simulink model "SF049A_LoaMgr"  (R2013b)
settings: Solver=FixedStepDiscrete  SolverMode=SingleTasking  StartTime=0.0  StopTime=1  FixedStep=0.002  RelTol=1e-3
undefined symbols (not defined in the file): CURRMEASLOAMTGTNMASK_CNT_U08, IVTRLOAMTGTNMASK_CNT_U08, LoaCtrldShtdwn, LoaCurrMeasIdptSigNrFlt, LoaHwTqIdptSigNrFlt, LoaImdtShtdwn, LoaIvtrIdptSigNrFlt, LOAMAXSLEW_ULSPERSEC_F32, LoaMgrCurrIvtrMtgtnRate, LoaMgrCurrIvtrMtgtnSca, LoaMgrCurrIvtrMtgtnScaZeroEna, LoaMgrCurrMeasIdptSig0Resp, LoaMgrCurrMeasIdptSig1Resp, LoaMgrCurrMeasIdptSig2Resp, LoaMgrCurrMeasIdptSigFltThd, LoaMgrCurrMeasMtgtnRate, LoaMgrCurrMeasMtgtnSca, LoaMgrCurrMeasMtgtnScaZeroEna, LoaMgrFadeOutStRate, LoaMgrHwTqIdptSig0NoTqLoaResp, LoaMgrHwTqIdptSig1NoTqLoaResp, LoaMgrHwTqIdptSig2Resp, LoaMgrHwTqIdptSig4Resp, LoaMgrHwTqIdptSigFltThd, LoaMgrHwTqLoaAvlResp, LoaMgrIvtrIdptSig0Resp, LoaMgrIvtrIdptSig1Resp, LoaMgrIvtrIdptSig2Resp, LoaMgrIvtrIdptSigFltThd, LoaMgrIvtrMtgtnRate, LoaMgrIvtrMtgtnSca, LoaMgrIvtrMtgtnScaZeroEna, LoaMgrLimdStRate, LoaMgrLimdStSca, LoaMgrMotAgAvlSnsrlsResp, LoaMgrMotAgIdptSig0NoSnsrlsResp, LoaMgrMotAgIdptSig1NoSnsrlsResp, LoaMgrMotAgIdptSig2Resp, LoaMgrMotAgIdptSig3Resp, LoaMgrMotAgIdptSigFltThd, LoaMgrMotAgMtgtnRate, LoaMgrMotAgMtgtnSca, LoaMgrMotAgMtgtnScaZeroEna, LoaMotAgIdptSigNrFlt, LOASCAONE_ULS_F32, LOASCAZERO_ULS_F32, LoaSt1, LOASTIMDTSHTDWN_CNT_U08, LOASTNORM_CNT_U08, LOASTSWMTGTN_CNT_U08, MAXCURRMEASIDPTSIGALLWD_CNT_U08, MAXHWTQIDPTSIGALLWD_CNT_U08, MAXIVTRIDPTSIGALLWD_CNT_U08, MAXMOTAGMECLIDPTSIGALLWD_CNT_U08, NODEBSTEP_CNT_U16, NtcSts1, SigQlfr1
libraries: simulink x30, NxtrMin x4, NxtrMax x4, NxtrLim x2
(part 7 of 7)

== system SF049A_LoaMgr/LoaMgr/LoaMgrPer1/Request_Responses/HwTqResp/Zero_or_Invalid/cal1 ==
  In1 : Inport
  Action Port : ActionPort  ActionType=then
  CopyRight2 : Subsystem  Description=|  mask(Copyright Information){none=on}
      | Copyright info block.                                               
      |                                                                     
      | Place copyright information at the top of every subsystem in design.
      mask prompts: none "No parameters"
      mask help: Place copyright information at the top of every subsystem in design.
      mask Display:
      | NxtrConf = 'Nexteer Confidential';
      | 
      | sys = bdroot; %handle for the current model ("system")
      | first = get_param(sys,'Created');
      | first = first(end-3:end);  %year is last four digits
      | 
      | last = get_param(sys,'LastModifiedDate');
      | if isempty(last)
      |     last = datestr(now,'yyyy');
      | else
      |     last = last(end-3:end);
      | end
      | 
      | if strcmp(first,last)
      |     fprintf('%s -- Copyright %s Nexteer',NxtrConf,first)
      | else
      |     fprintf('%s -- %s%s- %s Nexteer',NxtrConf,char(169),first,last)
      | end
  Out2 : Outport
  wires:
  In1/1 -> Out2/1

== system SF049A_LoaMgr/LoaMgr/LoaMgrPer1/Request_Responses/HwTqResp/Zero_or_Invalid/cal2 ==
  In1 : Inport
  Action Port : ActionPort  ActionType=else
  CopyRight2 : Subsystem  Description=|  mask(Copyright Information){none=on}
      | Copyright info block.                                               
      |                                                                     
      | Place copyright information at the top of every subsystem in design.
      mask prompts: none "No parameters"
      mask help: Place copyright information at the top of every subsystem in design.
      mask Display:
      | NxtrConf = 'Nexteer Confidential';
      | 
      | sys = bdroot; %handle for the current model ("system")
      | first = get_param(sys,'Created');
      | first = first(end-3:end);  %year is last four digits
      | 
      | last = get_param(sys,'LastModifiedDate');
      | if isempty(last)
      |     last = datestr(now,'yyyy');
      | else
      |     last = last(end-3:end);
      | end
      | 
      | if strcmp(first,last)
      |     fprintf('%s -- Copyright %s Nexteer',NxtrConf,first)
      | else
      |     fprintf('%s -- %s%s- %s Nexteer',NxtrConf,char(169),first,last)
      | end
  Out1 : Outport
  wires:
  In1/1 -> Out1/1

== system SF049A_LoaMgr/LoaMgr/LoaMgrPer1/Request_Responses/HwTqResp/one/CopyRight2 ==

== system SF049A_LoaMgr/LoaMgr/LoaMgrPer1/Request_Responses/HwTqResp/one/cal1 ==
  In1 : Inport
  Action Port : ActionPort  ActionType=then
  CopyRight2 : Subsystem  Description=|  mask(Copyright Information){none=on}
      | Copyright info block.                                               
      |                                                                     
      | Place copyright information at the top of every subsystem in design.
      mask prompts: none "No parameters"
      mask help: Place copyright information at the top of every subsystem in design.
      mask Display:
      | NxtrConf = 'Nexteer Confidential';
      | 
      | sys = bdroot; %handle for the current model ("system")
      | first = get_param(sys,'Created');
      | first = first(end-3:end);  %year is last four digits
      | 
      | last = get_param(sys,'LastModifiedDate');
      | if isempty(last)
      |     last = datestr(now,'yyyy');
      | else
      |     last = last(end-3:end);
      | end
      | 
      | if strcmp(first,last)
      |     fprintf('%s -- Copyright %s Nexteer',NxtrConf,first)
      | else
      |     fprintf('%s -- %s%s- %s Nexteer',NxtrConf,char(169),first,last)
      | end
  Out2 : Outport
  wires:
  In1/1 -> Out2/1

== system SF049A_LoaMgr/LoaMgr/LoaMgrPer1/Request_Responses/HwTqResp/one/cal2 ==
  In1 : Inport
  Action Port : ActionPort  ActionType=else
  CopyRight2 : Subsystem  Description=|  mask(Copyright Information){none=on}
      | Copyright info block.                                               
      |                                                                     
      | Place copyright information at the top of every subsystem in design.
      mask prompts: none "No parameters"
      mask help: Place copyright information at the top of every subsystem in design.
      mask Display:
      | NxtrConf = 'Nexteer Confidential';
      | 
      | sys = bdroot; %handle for the current model ("system")
      | first = get_param(sys,'Created');
      | first = first(end-3:end);  %year is last four digits
      | 
      | last = get_param(sys,'LastModifiedDate');
      | if isempty(last)
      |     last = datestr(now,'yyyy');
      | else
      |     last = last(end-3:end);
      | end
      | 
      | if strcmp(first,last)
      |     fprintf('%s -- Copyright %s Nexteer',NxtrConf,first)
      | else
      |     fprintf('%s -- %s%s- %s Nexteer',NxtrConf,char(169),first,last)
      | end
  Out1 : Outport
  wires:
  In1/1 -> Out1/1

== system SF049A_LoaMgr/LoaMgr/LoaMgrPer1/Request_Responses/InvtrResp/Two/CopyRight2 ==

== system SF049A_LoaMgr/LoaMgr/LoaMgrPer1/Request_Responses/InvtrResp/Zero_or_Invalid/CopyRight2 ==

== system SF049A_LoaMgr/LoaMgr/LoaMgrPer1/Request_Responses/InvtrResp/one/CopyRight2 ==

== system SF049A_LoaMgr/LoaMgr/LoaMgrPer1/Request_Responses/MotAgResp/Three/CopyRight2 ==

== system SF049A_LoaMgr/LoaMgr/LoaMgrPer1/Request_Responses/MotAgResp/Two/CopyRight2 ==

== system SF049A_LoaMgr/LoaMgr/LoaMgrPer1/Request_Responses/MotAgResp/Zero_or_Invalid/CopyRight2 ==

== system SF049A_LoaMgr/LoaMgr/LoaMgrPer1/Request_Responses/MotAgResp/Zero_or_Invalid/cal1 ==
  In1 : Inport
  Action Port : ActionPort  ActionType=then
  CopyRight2 : Subsystem  Description=|  mask(Copyright Information){none=on}
      | Copyright info block.                                               
      |                                                                     
      | Place copyright information at the top of every subsystem in design.
      mask prompts: none "No parameters"
      mask help: Place copyright information at the top of every subsystem in design.
      mask Display:
      | NxtrConf = 'Nexteer Confidential';
      | 
      | sys = bdroot; %handle for the current model ("system")
      | first = get_param(sys,'Created');
      | first = first(end-3:end);  %year is last four digits
      | 
      | last = get_param(sys,'LastModifiedDate');
      | if isempty(last)
      |     last = datestr(now,'yyyy');
      | else
      |     last = last(end-3:end);
      | end
      | 
      | if strcmp(first,last)
      |     fprintf('%s -- Copyright %s Nexteer',NxtrConf,first)
      | else
      |     fprintf('%s -- %s%s- %s Nexteer',NxtrConf,char(169),first,last)
      | end
  Out2 : Outport
  wires:
  In1/1 -> Out2/1

== system SF049A_LoaMgr/LoaMgr/LoaMgrPer1/Request_Responses/MotAgResp/Zero_or_Invalid/cal2 ==
  In1 : Inport
  Action Port : ActionPort  ActionType=else
  CopyRight2 : Subsystem  Description=|  mask(Copyright Information){none=on}
      | Copyright info block.                                               
      |                                                                     
      | Place copyright information at the top of every subsystem in design.
      mask prompts: none "No parameters"
      mask help: Place copyright information at the top of every subsystem in design.
      mask Display:
      | NxtrConf = 'Nexteer Confidential';
      | 
      | sys = bdroot; %handle for the current model ("system")
      | first = get_param(sys,'Created');
      | first = first(end-3:end);  %year is last four digits
      | 
      | last = get_param(sys,'LastModifiedDate');
      | if isempty(last)
      |     last = datestr(now,'yyyy');
      | else
      |     last = last(end-3:end);
      | end
      | 
      | if strcmp(first,last)
      |     fprintf('%s -- Copyright %s Nexteer',NxtrConf,first)
      | else
      |     fprintf('%s -- %s%s- %s Nexteer',NxtrConf,char(169),first,last)
      | end
  Out1 : Outport
  wires:
  In1/1 -> Out1/1

== system SF049A_LoaMgr/LoaMgr/LoaMgrPer1/Request_Responses/MotAgResp/one/CopyRight2 ==

== system SF049A_LoaMgr/LoaMgr/LoaMgrPer1/Request_Responses/MotAgResp/one/cal1 ==
  In1 : Inport
  Action Port : ActionPort  ActionType=then
  CopyRight2 : Subsystem  Description=|  mask(Copyright Information){none=on}
      | Copyright info block.                                               
      |                                                                     
      | Place copyright information at the top of every subsystem in design.
      mask prompts: none "No parameters"
      mask help: Place copyright information at the top of every subsystem in design.
      mask Display:
      | NxtrConf = 'Nexteer Confidential';
      | 
      | sys = bdroot; %handle for the current model ("system")
      | first = get_param(sys,'Created');
      | first = first(end-3:end);  %year is last four digits
      | 
      | last = get_param(sys,'LastModifiedDate');
      | if isempty(last)
      |     last = datestr(now,'yyyy');
      | else
      |     last = last(end-3:end);
      | end
      | 
      | if strcmp(first,last)
      |     fprintf('%s -- Copyright %s Nexteer',NxtrConf,first)
      | else
      |     fprintf('%s -- %s%s- %s Nexteer',NxtrConf,char(169),first,last)
      | end
  Out2 : Outport
  wires:
  In1/1 -> Out2/1

== system SF049A_LoaMgr/LoaMgr/LoaMgrPer1/Request_Responses/MotAgResp/one/cal2 ==
  In1 : Inport
  Action Port : ActionPort  ActionType=else
  CopyRight2 : Subsystem  Description=|  mask(Copyright Information){none=on}
      | Copyright info block.                                               
      |                                                                     
      | Place copyright information at the top of every subsystem in design.
      mask prompts: none "No parameters"
      mask help: Place copyright information at the top of every subsystem in design.
      mask Display:
      | NxtrConf = 'Nexteer Confidential';
      | 
      | sys = bdroot; %handle for the current model ("system")
      | first = get_param(sys,'Created');
      | first = first(end-3:end);  %year is last four digits
      | 
      | last = get_param(sys,'LastModifiedDate');
      | if isempty(last)
      |     last = datestr(now,'yyyy');
      | else
      |     last = last(end-3:end);
      | end
      | 
      | if strcmp(first,last)
      |     fprintf('%s -- Copyright %s Nexteer',NxtrConf,first)
      | else
      |     fprintf('%s -- %s%s- %s Nexteer',NxtrConf,char(169),first,last)
      | end
  Out1 : Outport
  wires:
  In1/1 -> Out1/1

== system SF049A_LoaMgr/LoaMgr/LoaMgrPer1/Set_Faults/NTC_Fault1/SetNtcSts/CopyRight2 ==

== system SF049A_LoaMgr/LoaMgr/LoaMgrPer1/Set_Faults/NTC_Fault2/SetNtcSts/CopyRight2 ==

== system SF049A_LoaMgr/LoaMgr/LoaMgrPer1/Set_Faults/NTC_Fault3/SetNtcSts/CopyRight2 ==

== system SF049A_LoaMgr/LoaMgr/LoaMgrPer1/Set_Faults/NTC_Fault4/SetNtcSts/CopyRight2 ==

== system SF049A_LoaMgr/LoaMgr/LoaMgrPer1/Assign_Scale/SwMtgtn/OthersTrue/CurrIvtr/CopyRight2 ==

== system SF049A_LoaMgr/LoaMgr/LoaMgrPer1/Assign_Scale/SwMtgtn/OthersTrue/CurrIvtr/PassThru1 ==
  In1 : Inport
  In2 : Inport  Port=2
  Action Port : ActionPort  ActionType=then
  Sca : Outport
  Rate : Outport  Port=2
  wires:
  In1/1 -> Sca/1
  In2/1 -> Rate/1

== system SF049A_LoaMgr/LoaMgr/LoaMgrPer1/Assign_Scale/SwMtgtn/OthersTrue/CurrIvtr/PassThru2 ==
  In1 : Inport
  In2 : Inport  Port=2
  Action Port : ActionPort  ActionType=else
  Sca : Outport
  Rate : Outport  Port=2
  wires:
  In1/1 -> Sca/1
  In2/1 -> Rate/1

== system SF049A_LoaMgr/LoaMgr/LoaMgrPer1/Assign_Scale/SwMtgtn/OthersTrue/CurrOnly/CopyRight2 ==

== system SF049A_LoaMgr/LoaMgr/LoaMgrPer1/Assign_Scale/SwMtgtn/OthersTrue/CurrOnly/PassThru1 ==
  In1 : Inport
  In2 : Inport  Port=2
  Action Port : ActionPort  ActionType=then
  Sca : Outport
  Rate : Outport  Port=2
  wires:
  In1/1 -> Sca/1
  In2/1 -> Rate/1

== system SF049A_LoaMgr/LoaMgr/LoaMgrPer1/Assign_Scale/SwMtgtn/OthersTrue/CurrOnly/PassThru2 ==
  In1 : Inport
  In2 : Inport  Port=2
  Action Port : ActionPort  ActionType=else
  Sca : Outport
  Rate : Outport  Port=2
  wires:
  In1/1 -> Sca/1
  In2/1 -> Rate/1

== system SF049A_LoaMgr/LoaMgr/LoaMgrPer1/Assign_Scale/SwMtgtn/OthersTrue/IvtrOnly/CopyRight2 ==

== system SF049A_LoaMgr/LoaMgr/LoaMgrPer1/Assign_Scale/SwMtgtn/OthersTrue/IvtrOnly/PassThru1 ==
  In1 : Inport
  In2 : Inport  Port=2
  Action Port : ActionPort  ActionType=then
  Sca : Outport
  Rate : Outport  Port=2
  wires:
  In1/1 -> Sca/1
  In2/1 -> Rate/1

== system SF049A_LoaMgr/LoaMgr/LoaMgrPer1/Assign_Scale/SwMtgtn/OthersTrue/IvtrOnly/PassThru2 ==
  In1 : Inport
  In2 : Inport  Port=2
  Action Port : ActionPort  ActionType=else
  Sca : Outport
  Rate : Outport  Port=2
  wires:
  In1/1 -> Sca/1
  In2/1 -> Rate/1

== system SF049A_LoaMgr/LoaMgr/LoaMgrPer1/Request_Responses/HwTqResp/Zero_or_Invalid/cal1/CopyRight2 ==

== system SF049A_LoaMgr/LoaMgr/LoaMgrPer1/Request_Responses/HwTqResp/Zero_or_Invalid/cal2/CopyRight2 ==

== system SF049A_LoaMgr/LoaMgr/LoaMgrPer1/Request_Responses/HwTqResp/one/cal1/CopyRight2 ==

== system SF049A_LoaMgr/LoaMgr/LoaMgrPer1/Request_Responses/HwTqResp/one/cal2/CopyRight2 ==

== system SF049A_LoaMgr/LoaMgr/LoaMgrPer1/Request_Responses/MotAgResp/Zero_or_Invalid/cal1/CopyRight2 ==

== system SF049A_LoaMgr/LoaMgr/LoaMgrPer1/Request_Responses/MotAgResp/Zero_or_Invalid/cal2/CopyRight2 ==

== system SF049A_LoaMgr/LoaMgr/LoaMgrPer1/Request_Responses/MotAgResp/one/cal1/CopyRight2 ==

== system SF049A_LoaMgr/LoaMgr/LoaMgrPer1/Request_Responses/MotAgResp/one/cal2/CopyRight2 ==
